simulink model "Sim_5_dead_signal"  (R2019b)
settings: Solver=VariableStepAuto  StartTime=0.0  StopTime=sim_time  FixedStep=0.01  MaxStep=0.1  MinStep=0.0001  RelTol=0.01  AbsTol=0.01
values from neighbouring files (symbols this model uses):
  Controller_Data = struct('K_p', K_p, 'K_v', K_v, 'K_i', K_i, 'M', M,     'D', D, 'U_ref', U_ref, 'mu', mu)    [Sim_10_init.m]    (also in Sim_11_init.m; Sim_12_init.m; Sim_3_4_and_5_init.m; Sim_7_8_userdef_init.m)
  D = [ 0.66  0    0 ... (first row only)    [Sim_10_init.m]    (also in Sim_11_init.m; Sim_12_init.m; Sim_3_4_and_5_init.m; Sim_7_8_userdef_init.m)
  K_p = 0.08*[1.1  0    0 ... (first row only)    [Sim_10_init.m]    (also in Sim_11_init.m; Sim_12_init.m; Sim_3_4_and_5_init.m; Sim_7_8_userdef_init.m)
  K_v = 1*[10   0       0 ... (first row only)    [Sim_10_init.m]    (also in Sim_11_init.m; Sim_12_init.m; Sim_3_4_and_5_init.m; Sim_7_8_userdef_init.m = 3*[10   0       0)
  LossOfSignalFalse = 1    [Sim_10_init.m]    (also in Sim_11_init.m; Sim_12_init.m; Sim_3_4_and_5_init.m; Sim_7_8_userdef_init.m)
  LossOfSignalTime = 10    [Sim_10_init.m]    (also in Sim_11_init.m; Sim_12_init.m; Sim_3_4_and_5_init.m = 30; Sim_7_8_userdef_init.m)
  LossOfSignalTrue = 0    [Sim_10_init.m]    (also in Sim_11_init.m; Sim_12_init.m; Sim_3_4_and_5_init.m; Sim_7_8_userdef_init.m)
  M = [ 16    0      0 ... (first row only)    [Sim_10_init.m]    (also in Sim_11_init.m; Sim_12_init.m; Sim_3_4_and_5_init.m; Sim_7_8_userdef_init.m)
  mu = 0.09    [Sim_10_init.m]    (also in Sim_11_init.m; Sim_12_init.m; Sim_3_4_and_5_init.m; Sim_7_8_userdef_init.m)
  Observergains = [L1, L2, L3]    [Sim_10_init.m]    (also in Sim_11_init.m; Sim_12_init.m; Sim_3_4_and_5_init.m; Sim_7_8_userdef_init.m)
  path_planner_data = [start_pos; end_pos; Radius; Center]    [Sim_10_init.m]    (also in Sim_11_init.m; Sim_12_init.m; Sim_3_4_and_5_init.m; Sim_7_8_userdef_init.m)
  pathparameter = 0    [Sim_10_init.m]    (also in Sim_11_init.m = 1; Sim_12_init.m; Sim_3_4_and_5_init.m = 1; Sim_7_8_userdef_init.m = 1)
  RegainOfSignalFalse = 0    [Sim_10_init.m]    (also in Sim_11_init.m; Sim_12_init.m; Sim_3_4_and_5_init.m; Sim_7_8_userdef_init.m)
  RegainOfSignalTime = 30    [Sim_10_init.m]    (also in Sim_11_init.m; Sim_12_init.m; Sim_3_4_and_5_init.m = 50; Sim_7_8_userdef_init.m)
  RegainOfSignalTrue = 1    [Sim_10_init.m]    (also in Sim_11_init.m; Sim_12_init.m; Sim_3_4_and_5_init.m; Sim_7_8_userdef_init.m)
  start_pos = [10; 20; pi/2 ]    [Sim_10_init.m]    (also in Sim_11_init.m = [0; 0; 0 ]; Sim_12_init.m = [0; 0; 0 ]; Sim_3_4_and_5_init.m = [0; 0; 0 ]; Sim_7_init.m = [0; 0; 0 ])
undefined symbols (not defined in the file or in its folder): eta_set, p, start_time, t1, t2, t3, time, tsamp, WP
(part 3 of 3)

== matlab function Sim_5_dead_signal/Controller/CtrlCustom_SLX/Backstepping controller/MATLAB Function ==
  data: eta input; path_planner_data output; tau_select output; clock_signal input; path_planner_data_in input; tau_select_in input; tau_ref output; start_pos input
function [path_planner_data, tau_select,tau_ref] = fcn(eta,clock_signal,path_planner_data_in,tau_select_in,start_pos)
%Straight-line
% start_pos = [0;0;0];
end_pos = [10;10;0];

%Elliptical
rx = 10;
ry = 20;
Cx = 0; %center of elipsoid
Cy = 0;

path_planner_data = [start_pos ; end_pos ; rx ; ry ; Cx ; Cy];
% path_planner_data = zeros(10,1);
tau_ref = [0.1;0.1;0.1];
tau_select = tau_select_in;
if clock_signal==50
    start_pos = [eta(1);eta(2);eta(3)];
    end_pos = [cos(eta(3))*200;sin(eta(3))*200;eta(3)];
    Cx = eta(1)-rx;
    Cy = eta(2);
    path_planner_data = [start_pos ; end_pos ; rx ; ry ; Cx ; Cy];
    tau_select = 1;
end

if clock_signal > 50
    path_planner_data = path_planner_data_in;
    

end

end

== matlab function Sim_5_dead_signal/Signal failure simulation, Dead reckoning function and Nonlinear Observer/MATLAB Function1 ==
  settings: updateMethod=DISCRETE
  data: eta input size=3; eta_out output size=3; deadreckoning output; prev_eta input; LoS_check input; stored_eta output
function [eta_out, deadreckoning, stored_eta] = Deadreck(eta, prev_eta,  LoS_check)

    if not(LoS_check) %If loss of signal is true, i.e LoS_check = 0
        dead_signal = true;
        for i = 1:3 %Check if current measurement and 3 prior positions are equal
            if eta ~= prev_eta(i,:)'
              dead_signal = false;
            end
        end
          
        if dead_signal %If four last signal values are equal, set output to be equal to eta_hat when we last had 
            deadreckoning = 1;
            eta_out = eta;

        else %Signal is not dead or frozen - Do normal stuff
            deadreckoning = 1;
            eta_out = eta;

        end
    else %If measurements are available - Do normal stuff
        deadreckoning = 0;
        eta_out = eta;
    end

stored_eta = prev_eta;
stored_eta(1:2,:) = prev_eta(end-1:end,:);
stored_eta(end,:) = eta';
end

== matlab function Sim_5_dead_signal/Signal failure simulation, Dead reckoning function and Nonlinear Observer/Nonlinear Observer ==
  settings: updateMethod=DISCRETE
  data: eta input; eta_hat input; nu_hat input; b_hat input; eta_hat_dot output size=3; DR input; tau input; nu_hat_dot output size=3; Observergains parameter; Controller_Data parameter; b_hat_dot output size=3; eta_tilde output
function [eta_hat_dot, nu_hat_dot, b_hat_dot, eta_tilde] = Nonlinear_Observer(eta, eta_hat, nu_hat, b_hat,DR, tau, Observergains, Controller_Data)

persistent M D
    [M, D] = deal(Controller_Data.M, Controller_Data.D);

scaling = 0.01/0.1;
L1 = scaling*Observergains(1:3,1:3);
L2 = scaling*Observergains(1:3,4:6);
L3 = scaling*Observergains(1:3,7:9);

psi = eta(3,1);

if DR
    L1 = 0*L1;
    L2 = 0*L2;
    L3 = 0*L3;
    psi = eta_hat(3,1);
end

R_psi = [ cos(psi)  -sin(psi)   0  ;
          sin(psi)    cos(psi)  0  ; 
          0              0         1  ] ;
R_tr = transpose(R_psi);

eta_tilde = eta - eta_hat;

eta_hat_dot = R_psi*nu_hat + L1*eta_tilde;
nu_hat_dot = M\(-D*nu_hat + R_tr*b_hat + tau + R_tr*L2*eta_tilde);
b_hat_dot = L3*eta_tilde;

end

== matlab function Sim_5_dead_signal/Wrap2QualisysOutput 1/Wrap2psi ==
  data: u input; yQualisus output
function yQualisus = fcn(u)
y=sin(u);
x=cos(u);
yQualisus=atan2(y,x);
end

== matlab function Sim_5_dead_signal/Signal failure simulation, Dead reckoning function and Nonlinear Observer/Pose1/MATLAB Function ==
  data: psi input; psi_out output; psi_old input
function psi_out = fcn(psi,psi_old)
psi_out=psi_old+angdiff(psi_old,psi);

== matlab function Sim_5_dead_signal/Signal failure simulation, Dead reckoning function and Nonlinear Observer/Simlate a loss of signal function ==
  settings: updateMethod=DISCRETE
  data: eta_measured input size=3; eta_out output size=3; LossOfSignalValue output; Loss_of_signal_detection input; prior_measurement_in input; prior_measurement_out output
function [eta_out, LossOfSignalValue, prior_measurement_out] = SimLoS(eta_measured, Loss_of_signal_detection, prior_measurement_in)

% Simulates a loss of signal/frozen signal, where it keeps sending out the
% same measurement while the LossOfSignalDetection returns 0 as stated in
% task 4.4 and 4.5 from case B

    if not(Loss_of_signal_detection)
        eta_out = prior_measurement_in;
        prior_measurement_out = prior_measurement_in;
        LossOfSignalValue = Loss_of_signal_detection;
        
    else
        eta_out = eta_measured;
        prior_measurement_out = eta_measured;
        LossOfSignalValue = Loss_of_signal_detection;
    end
end

== matlab function Sim_5_dead_signal/Controller/CtrlCustom_SLX/Backstepping controller/Rotation Matrix ==
  data: psi input; R_psi output
function R_psi = fcn(psi)
R_psi = [ cos(psi)  -sin(psi)   0  ;
                sin(psi)    cos(psi)  0  ; 
                    0              0         1  ] ;
end

== matlab function Sim_5_dead_signal/Controller/CtrlCustom_SLX/Backstepping controller/Sideslip compensation /LOS Lookahead Guidance ==
  data: p input; chi_d output size=1; WP input; segment_switch_lookahead_dist parameter; s input; track input; e_x output; e_y output
function [chi_d, e_x, e_y] = straight_line_path_handler(p, WP, segment_switch_lookahead_dist, s, track)

persistent current_segment;

if isempty(current_segment)
    current_segment = 1;
end

path_lookahead_dist = 0.5*segment_switch_lookahead_dist;

if not(track)
    p0 = WP(:,current_segment); % start wp in current segment
    p1 = WP(:, current_segment+1); % end wp in current segment
    num_segments = size(WP);
    num_segments = num_segments(2);

% update segment
% if next wp is closer to boat than path_lookahead_dist
% and not on last segment
    d_next_wp = p1 - p;
    d_next_wp = sqrt(dot(d_next_wp, d_next_wp));
    if current_segment + 1 < num_segments && d_next_wp <= segment_switch_lookahead_dist
        current_segment = current_segment + 1; 
        p0 = WP(:,current_segment);
        p1 = WP(:, current_segment+1);
    end
    % get path tangential angle
    % get x track and along track err
    alpha_k = atan2( p1(2) - p0(2), p1(1) - p0(1));
else
    % track
    p0 = WP(:,1); % start wp in current segment
    p1 = WP(:,2); % end wp in current segment
    alpha_k = atan2( p1(2) - p0(2), p1(1) - p0(1));
%     alpha_k
    p1(1) = p1(1) + s*3*cos(alpha_k);
    p1(2) = p1(2) + s*3*sin(alpha_k);
end

% current_segment = current_segment+1;
% cross track error
e_x = -(p(1) - p1(1))*sin(alpha_k) + (p(2) - p1(2))*cos(alpha_k);
% along track error
e_y = (p(1) - p1(1))*cos(alpha_k) + (p(2) - p1(2))*sin(alpha_k);
% lookahead based steering
chi_p = alpha_k;
%tan_chi_r = -e_x / path_lookahead_dist;
chi_r = atan(-e_x / path_lookahead_dist);
chi_d = chi_p + chi_r;

== matlab function Sim_5_dead_signal/Controller/CtrlCustom_SLX/Backstepping controller/Sideslip compensation /Course calculation ==
  settings: updateMethod=DISCRETE
  data: p input; chi output size=1
function chi = compute_chi(p)

persistent p_prev;

if isempty(p_prev)
    p_prev = p;
    chi = 0;
else
    dy = p(2) - p_prev(2);
    dx = p(1) - p_prev(1);
    p_prev = p;
    chi = atan2(dy, dx);
    if chi < 0
        chi = chi + 2*pi;
    end
end

== matlab function Sim_5_dead_signal/Controller/CtrlCustom_SLX/Backstepping controller/S(psi_dot) ==
  data: r input; S_r output
function S_r = fcn(r)
S_r = [ 0  -r   0  ;
         r  0   0   ; 
         0  0   1  ] ;
end

== matlab function Sim_5_dead_signal/Controller/CtrlCustom_SLX/Backstepping controller/Transpose Rotation Matrix ==
  data: psi input; R_psi_trans output
function R_psi_trans = fcn(psi)
R_psi = [ cos(psi)  -sin(psi)   0  ;
                sin(psi)    cos(psi)  0  ; 
                    0              0         1  ] ;
                
R_psi_trans = transpose(R_psi);
end

== matlab function Sim_5_dead_signal/Controller/CtrlCustom_SLX/Backstepping controller/Sideslip compensation /MATLAB Function1 ==
  data: psi input; psi_ref input; psi_ref_new output
function psi_ref_new = ssa( psi, psi_ref)

val1 = psi_ref;
val2 = psi_ref + 2*pi;
val3 = psi_ref - 2*pi;

vals = [val1, val2, val3];

[m, i] = min(abs(vals - psi));

psi_ref_new = vals(i);

== matlab function Sim_5_dead_signal/Controller/CtrlCustom_SLX/Transpose Rotation Matrix ==
  data: psi input; R_psi_trans output
function R_psi_trans = fcn(psi)
R_psi = [ cos(psi)  -sin(psi)   0  ;
                sin(psi)    cos(psi)  0  ; 
                    0              0         1  ] ;
                
R_psi_trans = transpose(R_psi);
end

== matlab function Sim_5_dead_signal/Controller/CtrlCustom_SLX/Backstepping controller/alpha1, z_1 explicit ==
  data: alpha_1 output; eta_d input; eta_df input; eta input; s_dot input; nu_hat input; z_1 output
function [alpha_1, z_1] = fcn(eta_d, eta_df, eta, s_dot, nu_hat)

psi = eta(3);
r = nu_hat(3);

R_psi = [ cos(psi)  -sin(psi)   0  ;
                sin(psi)    cos(psi)  0  ; 
                    0              0         1  ] ;
R_transp = transpose(R_psi);
                
S_r = [ 0  -r   0  ;
         r  0   0   ; 
         0  0   1  ] ;   

[alpha_1, z_1] = -S_r*R_transp*(eta - eta_d) + nu_hat - R_transp*eta_df*s_dot;

== matlab function Sim_5_dead_signal/Controller/CtrlCustom_SLX/Backstepping controller/alpha_1, z_1 - explicit /Rotation Matrix ==
  data: psi input; R_psi output
function R_psi = fcn(psi)
R_psi = [ cos(psi)  -sin(psi)   0  ;
                sin(psi)    cos(psi)  0  ; 
                    0              0         1  ] ;
end

== matlab function Sim_5_dead_signal/Controller/CtrlCustom_SLX/Backstepping controller/d//dt[....] ==
  data: eta input; eta_df input; d_dt output size=3; eta_dff input; nu_hat input; s_dot input; U_s input; U_sf input
function d_dt = fcn(eta, eta_df, eta_dff, nu_hat, s_dot, U_s, U_sf)

psi = eta(3);
r = nu_hat(3);

R_psi = [ cos(psi)  -sin(psi)   0  ;
                sin(psi)    cos(psi)  0  ; 
                    0              0         1  ] ;
R_tr = transpose(R_psi);
                
S_r = [ 0  -r   0  ;
         r  0   0   ; 
         0  0   0  ] ;
     
S_tr = transpose(S_r);

d_dt = S_tr*R_tr*eta_df*U_s + R_tr*s_dot*(eta_dff*U_s + eta_df*U_sf);

== matlab function Sim_5_dead_signal/Controller/CtrlCustom_SLX/Backstepping controller/z_1_dot ==
  data: z_1_dot output size=3; eta_d input; eta_df input; eta input; s_dot input; nu_hat input
function z_1_dot = fcn(eta_d, eta_df, eta, s_dot, nu_hat)

psi = eta(3);
r = nu_hat(3);

R_psi = [ cos(psi)  -sin(psi)   0  ;
                sin(psi)    cos(psi)  0  ; 
                    0              0         1  ] ;
R_transp = transpose(R_psi);
                
S_r = [ 0  -r   0  ;
         r  0   0   ; 
         0  0  0   ] ;   

z_1_dot = -S_r*R_transp*(eta - eta_d) + nu_hat - R_transp*eta_df*s_dot;
